simulink model "hexa_tilted_PID"  (R2023a)
settings: Solver=ode4  StartTime=0.0  StopTime=10  FixedStep=0.01  RelTol=1e-3
model workspace (MAT data in the model file):
  tf = Simulink.Parameter
  tf.Value = 60
  tf.DataType = 'auto'
  tf.Complexity = 'real'
  tf.Dimensions = [1 1]
  tray1 = [0  0  0  0  0  0; 0  0  0  0  0  0; 0  2  2  2  2  0; 0  0  0  0  0  0; 0  0  0  0  0  0; 0  0  0  0  0  0]
  tray2 = [0  2  2  -2  0  0; 0  -2  -2  2  0  0; 0  2  2  2  2  0; 0  0  0  0  0  0; 0  0  0  0  0  0; 0  0  0  0  0  0]
libraries: dspsrcs4 x6, simulink x3, robotcorelib x1
settings Model: Creator=adan  LastModifiedBy=adan
settings OptimizationCC: ReuseModelBlockBuffer=off

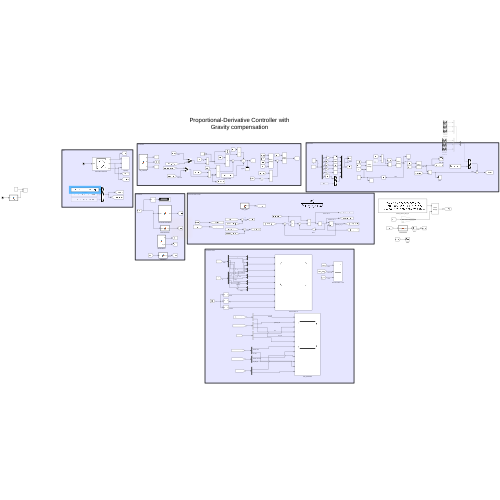
[thumbnail: Simulink's stored preview of the top-level diagram]
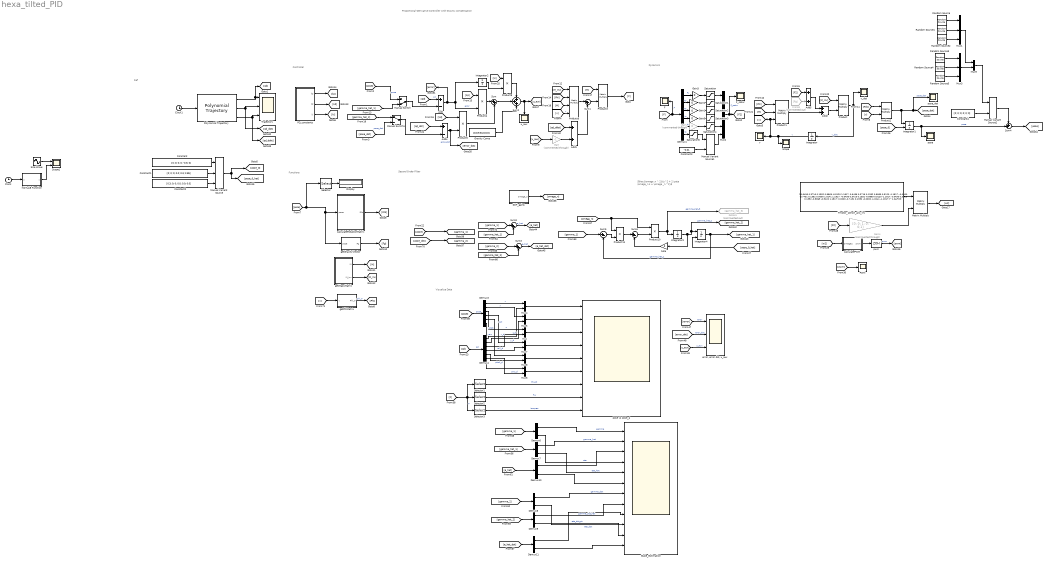
== system hexa_tilted_PID ==
  note: Ref
  note: Functions
  note: Second Order Filter
  note: Controller
  note: Visualize Data
  note: Dynamics
  note: Proportional-Derivative Controller with Gravity compensation
  note: $\frac{\omega_n ^ 2}{s^2 + 2 \zeta \omega_n s + \omega _n ^2}$
  Add : Sum  Inputs=+-
  Add1 : Sum
  Add2 : Sum
  Add4 : Sum  Inputs=+-
  Add5 : Sum
  Clock : Clock
  Clock1 : Clock
  Constant : Constant  Value=[0; 0; 0; 0; -0.3; 0]
  Constant1 : Constant  Value=[0; 0; 0; 0.0; 0.3; 2.85]
  Constant2 : Constant  Value=[0.3; 0; 0; 0.0; 0.0; 0.0]
  Constant3 : Constant  Value=-0.01
  Constant4 : Constant  Value=[0; 0; 0; 0; 0; 0]
  Demux1 : Demux  Outputs=6
  Demux{6..11} (6 alike) : Demux  Outputs=2
  Demux3 : Demux  Outputs=6
  Demux4 : Demux  Outputs=6
  Display : Display
  F : Scope
  F_satur : Scope
  From8 : From  Commented=on  GotoTag=Fg
  Gain : Gain  Commented=through  Gain=-1
  Gain{1..3,5} (4 alike) : Gain  Gain=0
  Gain4 : Gain  Commented=through  Gain=[0; 0; 1; 0; 0;1]
  Gain6 : Gain  Commented=through  Gain=0
  Goto41 : Goto  Commented=on  GotoTag=gamma_hat_3
  Gravity Comp : Constant  Value=[0;0;9.81;0;0;0]
  Integrator : Integrator  InitialCondition=[0; 0; 0; 0; 0; 0]
  Integrator1 : Integrator  InitialConditionSource=external  InitialCondition=[0; 0; 0; 0; 0; 0]
  Integrator2 : Integrator
  Integrator3 : Integrator
  Integrator4 : Integrator  InitialConditionSource=external
  MATLAB Function : MATLAB Function  TreatAsAtomicUnit=on
  Manual Variant Source : simulink/Signal Routing/Manual Variant Source  NumChoices=3  LabelModeActiveChoice=V_1
  Manual Variant Source1 : simulink/Signal Routing/Manual Variant Source  NumChoices=2  LabelModeActiveChoice=V_1
  Manual Variant Source2 : simulink/Signal Routing/Manual Variant Source  NumChoices=2  LabelModeActiveChoice=V_2
  Manual Switch : ManualSwitch  CurrentSetting=0
  Manual Switch1 : ManualSwitch
  Matrix Multiply : Product  Multiplication=Matrix(*)
  Mux{,4..9} (7 alike) : Mux  Inputs=2
  Mux1 : Mux  Inputs=3
  Mux2 : Mux  Inputs=6
  Mux3 : Mux  Inputs=3
  PD_constants : MATLAB Function  TreatAsAtomicUnit=on
  PWM : Scope
  Polynomial Trajectory : robotcorelib/Polynomial Trajectory  WaypointSource=Internal  Waypoints=zeros(6, 6)  TimePoints=[ 0, 5, 20, 28, 54, tf ]  TimeInterval=[ 1, 4 ]  Method=Cubic Polynomial  ParameterSource=Internal  VelocityBoundaryCondition=zeros( 6, 6 )  AccelerationBoundaryCondition=zeros( 2, 5 )  SimulateUsing=Interpreted execution
  Product : Product  Multiplication=Matrix(*)
  Product1 : Product  Inputs=3  Multiplication=Matrix(*)
  Product{4..5,8,10..11} (5 alike) : Product
  Product2 : Product  Multiplication=Matrix(*)
  Product3 : Product  Multiplication=Matrix(*)
  Product6 : Product  Inputs=4  Multiplication=Matrix(*)
  Random Source : dspsrcs4/Random Source  SrcType=Gaussian  NormMethod=Ziggurat  CltLength=12  MinVal=0  MaxVal=1  MeanVal=0.005  VarVal=0.001*0.001  RepMode=Not repeatable  rawSeed=1  IsInherit=off  SampMode=Discrete  SampTime=0.01  SampFrame=1  DataType=Double  OutComplex=Real  OutputFrames=off
  Random Source1 : dspsrcs4/Random Source  SrcType=Gaussian  NormMethod=Ziggurat  CltLength=12  MinVal=0  MaxVal=1  MeanVal=0.005  VarVal=0.001*0.001  RepMode=Not repeatable  rawSeed=1  IsInherit=off  SampMode=Discrete  SampTime=0.01  SampFrame=1  DataType=Double  OutComplex=Real  OutputFrames=off
  Random Source2 : dspsrcs4/Random Source  SrcType=Gaussian  NormMethod=Ziggurat  CltLength=12  MinVal=0  MaxVal=1  MeanVal=0.005  VarVal=0.001*0.001  RepMode=Not repeatable  rawSeed=1  IsInherit=off  SampMode=Discrete  SampTime=0.01  SampFrame=1  DataType=Double  OutComplex=Real  OutputFrames=off
  Random Source3 : dspsrcs4/Random Source  SrcType=Gaussian  NormMethod=Ziggurat  CltLength=12  MinVal=0  MaxVal=1  MeanVal=0.001  VarVal=0.001*0.001  RepMode=Not repeatable  rawSeed=1  IsInherit=off  SampMode=Discrete  SampTime=0.01  SampFrame=1  DataType=Double  OutComplex=Real  OutputFrames=off
  Random Source4 : dspsrcs4/Random Source  SrcType=Gaussian  NormMethod=Ziggurat  CltLength=12  MinVal=0  MaxVal=1  MeanVal=0.001  VarVal=0.001*0.001  RepMode=Not repeatable  rawSeed=1  IsInherit=off  SampMode=Discrete  SampTime=0.01  SampFrame=1  DataType=Double  OutComplex=Real  OutputFrames=off
  Random Source5 : dspsrcs4/Random Source  SrcType=Gaussian  NormMethod=Ziggurat  CltLength=12  MinVal=0  MaxVal=1  MeanVal=0.001  VarVal=0.001*0.001  RepMode=Not repeatable  rawSeed=1  IsInherit=off  SampMode=Discrete  SampTime=0.01  SampFrame=1  DataType=Double  OutComplex=Real  OutputFrames=off
  SOF_gains : MATLAB Function  TreatAsAtomicUnit=on
  Saturation : Saturate  UpperLimit=6  LowerLimit=-6
  Saturation1 : Saturate  UpperLimit=6  LowerLimit=-6
  Saturation2 : Saturate  UpperLimit=35  LowerLimit=0
  Saturation3 : Saturate
  Saturation4 : Saturate
  Saturation5 : Saturate
  Scope : Scope
  Scope1 : Scope  NumInputPorts=2
  Selector : Selector  InputPortWidth=6  IndexOptions=Index vector (dialog)  Indices=[4]  OutputSizes=1
  Selector1 : Selector  InputPortWidth=6  IndexOptions=Index vector (dialog)  Indices=[3]  OutputSizes=1
  Selector2 : Selector  InputPortWidth=6  IndexOptions=Index vector (dialog)  Indices=[1:2]  OutputSizes=1
  Selector3 : Selector  InputPortWidth=6  IndexOptions=Index vector (dialog)  Indices=[4:6]  OutputSizes=1
  Sine Wave : Sin  Amplitude=0.25  Frequency=0.5  SampleTime=0
  State_Estimation : Scope  NumInputPorts=12
  Sum : Sum  Inputs=|++
  Sum1 : Sum  Inputs=|-+
  Sum2 : Sum  Inputs=+++
  Sum{3,5..6,8} (4 alike) : Sum  Inputs=|+-
  Sum4 : Sum  Inputs=++|
  Tmotor_10inch_allo_inv : Constant  Value=|
      | [-0.6436    0.3716    0.1352    0.8869   -0.5120    1.1817;
      |             0.6436    0.3716    0.1352    0.8869    0.5120   -1.1817;
      |             -0.0000   -0.7431    0.1352    0.0000    1.0241    1.1817;
      |             -0.6436    0.3716    0.1352   -0.8869    0.5120   -1.1817;
      |             0.6436    0.3716    0.1352   -0.8869   -0.5120    1.1817;
      |             0.0000   -0.7431    0.1352   -0.0000   -1.0241   -1.1817;] * 1.0e+05;
  Trajectory : Scope  NumInputPorts=3
  calculatePWM : MATLAB Function  TreatAsAtomicUnit=on
  calculateRotationMatrix : MATLAB Function  TreatAsAtomicUnit=on
  "error, error dot, u_aux" : Scope  NumInputPorts=3
  getGravityVector : MATLAB Function  TreatAsAtomicUnit=on
  getMassMatrix : MATLAB Function  TreatAsAtomicUnit=on
  getPhiMatrix : MATLAB Function  TreatAsAtomicUnit=on
  pose : Scope
  pose vs pose_q : Scope  NumInputPorts=9
  pose_dot : Scope
  pwm : ZeroOrderHold  SampleTime=-1
  u_aux : Scope
  v : Scope
  v_dot : Scope
  zeta : Gain  Gain=2
  wires:
  Saturation/1 -> Mux2/1
  Saturation1/1 -> Mux2/2
  Saturation4/1 -> Mux2/5
  Saturation3/1 -> Mux2/4
  Demux1/6 -> Saturation5/1  "tz"
  Demux1/3 -> Gain1/1  "Fz"
  [F] -> F/1, Demux1/1  "F"
  Saturation5/1 -> Manual Variant Source1/1
  Demux1/2 -> Gain2/1  "Fy"
  Demux1/1 -> Gain3/1  "Fx"
  Demux1/5 -> Gain6/1  "ty"
  Demux1/4 -> Gain5/1  "tx"
  Saturation2/1 -> Mux2/3
  Mux2/1 -> F_satur/1, [F2]  "F_satur"
  [M] -> Product1/2
  [v] -> Product2/2
  [M_inv] -> Product/1
  Add2/1 -> Product/2
  Product/1 -> v_dot/1, Integrator/1  "v_dot"
  [Rib] -> Product2/1
  Product2/1 -> pose_dot/1, [pose_dot], Integrator1/1  "pose_dot"
  [Phi] -> Product1/1
  Product1/1 -> Add2/2
  Integrator1/1 -> pose/1, Sum4/2  "pose"
  Integrator/1 -> Scope/1, v/1, [v], Product1/3  "v"
  From8/1 -> Add5/2
  Add5/1 -> Add2/1
  [pose_dot] -> Manual Switch1/2  "pose_dot"
  [qd_dot] -> Add4/1
  [Phi] -> Product6/2
  Add4/1 -> [error_dot], Product5/2  "error_dot"
  [qd_ddot] -> Add1/1
  [qd] -> Add/1  "xd"
  [kp] -> Product4/1
  [v] -> Product6/4  "v"
  [kd] -> Product5/1
  Product4/1 -> Sum/1
  [M_inv] -> Product6/1
  [M] -> Product6/3
  Add/1 -> [error], Product4/2, Integrator2/1  "error"
  Product5/1 -> Sum/2
  [u_aux] -> Gain/1
  Sum2/1 -> [u_aux], u_aux/1
  [F2] -> Add5/1
  [ki] -> Product8/1
  Integrator2/1 -> Product8/2
  Gravity Comp/1 -> Sum2/3
  Sum/1 -> Sum2/2
  Product8/1 -> Sum2/1
  Add1/1 -> Sum1/2
  calculateRotationMatrix/1(Rib) -> [Rib]
  [pose] -> Selector/1, getGravityVector/1(pose), calculateRotationMatrix/1(pose)
  getGravityVector/1(Fg) -> [Fg]
  getPhiMatrix/1(Phi_T) -> [Phi]  "phi_T"
  Clock1/1 -> Polynomial Trajectory/1
  Polynomial Trajectory/2 -> Trajectory/2, [qd_dot]
  Polynomial Trajectory/3 -> Trajectory/3, [qd_ddot]
  Polynomial Trajectory/1 -> [qd], Trajectory/1
  Product6/1 -> Sum1/1
  Sum1/1 -> Product3/2
  [M] -> Product3/1
  Product3/1 -> [F]
  Demux3/5 -> Mux8/1  "pitch"
  Demux4/4 -> Mux7/2  "roll_d"
  Demux3/2 -> Mux5/1  "y"
  Mux5/1 -> pose vs pose_q/2
  Demux3/3 -> Mux/1  "z"
  [qd] -> Demux4/1  "qd"
  Mux8/1 -> pose vs pose_q/5
  Mux7/1 -> pose vs pose_q/4
  Mux4/1 -> pose vs pose_q/1
  Demux4/6 -> Mux6/2  "yaw_d"
  Demux4/1 -> Mux4/2  "x_d"
  Demux3/1 -> Mux4/1  "x"
  Demux3/4 -> Mux7/1  "roll"
  Mux6/1 -> pose vs pose_q/6
  [pose] -> Demux3/1  "pose"
  Mux/1 -> pose vs pose_q/3
  Demux4/5 -> Mux8/2  "pitch_d"
  Demux4/3 -> Mux/2  "z_d"
  Demux3/6 -> Mux6/1  "yaw"
  Demux4/2 -> Mux5/2  "y_d"
  [error_dot] -> "error, error dot, u_aux"/2  "error_dot"
  [error] -> "error, error dot, u_aux"/1  "error"
  [u_aux] -> "error, error dot, u_aux"/3  "u_aux"
  [gamma_hat_2] -> Demux9/1
  [gamma_hat_1] -> Demux7/1
  Demux6/2 -> State_Estimation/4  "eta"
  Demux7/2 -> State_Estimation/5  "eta_hat"
  Demux8/2 -> State_Estimation/10  "eta_dot"
  [gamma_2] -> Sum3/1
  [gamma_2] -> Demux8/1
  [omega_n] -> Product11/1, Product10/1
  [gamma_1] -> Demux6/1
  [e_hat_dot] -> Demux11/1
  Demux8/1 -> State_Estimation/7  "gamma_dot"
  SOF_gains/1(omega_n) -> [omega_n]
  [gamma_hat_2] -> Sum3/2
  [gamma_1] -> Sum8/1
  Demux11/1 -> State_Estimation/9
  Integrator3/1 -> zeta/1, [gamma_hat_2], Integrator4/1  "gamma_hat_2"
  Demux6/1 -> State_Estimation/1  "gamma"
  [gamma_1] -> Sum5/1
  Demux9/2 -> State_Estimation/11  "eta_dot_at"
  zeta/1 -> Sum6/2
  Demux11/2 -> State_Estimation/12
  Demux10/2 -> State_Estimation/6
  [e_hat] -> Demux10/1
  Demux7/1 -> State_Estimation/2  "gamma_hat"
  Demux10/1 -> State_Estimation/3
  Sum6/1 -> Product10/2
  Sum3/1 -> [e_hat_dot]  "e_hat"
  Integrator4/1 -> Sum5/2, [gamma_hat_1]  "gamma_hat_1"
  Sum5/1 -> Product11/2
  [gamma_hat_1] -> Sum8/2
  Sum8/1 -> [e_hat]  "e_hat"
  Product10/1 -> Integrator3/1, Goto41/1  "gamma_hat_3"
  Product11/1 -> Sum6/1
  Demux9/1 -> State_Estimation/8  "gamma_dot_hat"
  [pose] -> [gamma_1]
  [pose_dot] -> [gamma_2]
  PD_constants/3(ki) -> [ki]
  [v] -> getPhiMatrix/1(v)
  getMassMatrix/2(M_inv) -> [M_inv]
  getMassMatrix/1(M) -> [M]
  Gain/1 -> Add1/2
  [pose] -> Manual Switch/1  "pose"
  [gamma_hat_1] -> Manual Switch/2
  Manual Switch/1 -> Add/2
  [gamma_hat_2] -> Manual Switch1/1
  Manual Switch1/1 -> Add4/2
  Selector/1 -> Display/1
  Constant/1 -> Manual Variant Source/1
  Constant1/1 -> Manual Variant Source/2
  Manual Variant Source/1 -> [pose_0], [pose_0_hat]
  [pose_0] -> Integrator1/2
  [pose_0_hat] -> Integrator4/2
  [F] -> Selector1/1, Selector3/1, Selector2/1  "F"
  Selector1/1 -> pose vs pose_q/7  "thrust"
  Selector2/1 -> pose vs pose_q/8  "fxy"
  Selector3/1 -> pose vs pose_q/9  "torques"
  PD_constants/1(kp) -> [kp]
  PD_constants/2(kd) -> [kd]
  Constant2/1 -> Manual Variant Source/3
  Gain1/1 -> Saturation2/1
  Gain2/1 -> Saturation1/1
  Gain3/1 -> Saturation/1
  Tmotor_10inch_allo_inv/1 -> Matrix Multiply/1
  [F2] -> Gain4/1
  calculatePWM/1(pwm) -> pwm/1
  [w2] -> calculatePWM/1(omega2)
  [pwm] -> PWM/1
  pwm/1 -> [pwm]  "pwm"
  Matrix Multiply/1 -> [w2]
  Gain4/1 -> Matrix Multiply/2
  Gain5/1 -> Saturation3/1
  Gain6/1 -> Saturation4/1
  Manual Variant Source1/1 -> Mux2/6
  Constant3/1 -> Manual Variant Source1/2
  Sine Wave/1 -> Scope1/1
  Clock/1 -> MATLAB Function/1(u)
  MATLAB Function/1(y) -> Scope1/2
  Sum4/1 -> [pose]
  Manual Variant Source2/1 -> Sum4/1
  Constant4/1 -> Manual Variant Source2/2
  Random Source/1 -> Mux1/1
  Random Source2/1 -> Mux1/3
  Random Source1/1 -> Mux1/2
  Random Source4/1 -> Mux3/2
  Random Source5/1 -> Mux3/3
  Random Source3/1 -> Mux3/1
  Mux3/1 -> Mux9/2
  Mux1/1 -> Mux9/1
  Mux9/1 -> Manual Variant Source2/1

== matlab function hexa_tilted_PID/getPhiMatrix ==
  data: v input; Phi_T output
function Phi_T = fcn(v)

%% Phi matrix calculation
uu = v(1);
vv = v(2);
ww = v(3);
pp = v(4);
qq = v(5);
rr = v(6);


Phi = [0, -rr, qq, 0, -ww, vv;
        rr, 0, -pp , ww, 0, -uu;
        -qq, pp, 0,  -vv, uu, 0;
        0, 0, 0, 0, -rr, qq; 
        0, 0, 0, rr, 0, -pp;
        0, 0, 0, -qq, pp, 0];

Phi_T = Phi;

== matlab function hexa_tilted_PID/PD_constants ==
  data: kp output; kd output; ki output
function [kp, kd, ki] = fcn

%% Buenas ganancias
% kp = [3.5; 3.5; 3; 1.1; 1.1; 0.85];
% kd = [3.25; 3.25; 3; 1.75; 1.75; 1.5];

%% Ganancias lentas
kp = [0.1; 0.1; 0.01; 0.05; 2; 2];
kd = [0.5; 0.5; 0.2; 0.5; 2; 2];
ki = [0; 0; 0; 0; 0; 0];

== matlab function hexa_tilted_PID/calculateRotationMatrix ==
  data: Rib output; pose input
function Rib  = fcn(pose)

roll = pose(4);
pitch = pose(5);
yaw = pose(6);

R1 = [cos(yaw)*cos(pitch), -cos(roll)*sin(yaw) + cos(yaw)*sin(roll)*sin(pitch), sin(roll)*sin(yaw) + cos(roll)*cos(yaw)*sin(pitch);
       cos(pitch)*sin(yaw), cos(roll)*cos(yaw) + sin(yaw)*sin(pitch)*sin(roll), -cos(yaw)*sin(roll) + sin(yaw)*sin(pitch)*cos(roll);
       -sin(pitch), cos(pitch)*sin(roll), cos(pitch)*cos(roll)];

R2 = [1, sin(roll)*tan(pitch), cos(roll)*tan(pitch);
      0, cos(roll), -sin(roll);
      0, sin(roll)/cos(pitch), cos(roll)/cos(pitch)];

Rzeros = zeros(3);

Rib = [R1, Rzeros;
       Rzeros, R2];

== matlab function hexa_tilted_PID/getMassMatrix ==
  data: M output; M_inv output
function [M, M_inv] = fcn

m = 1.8;
Jxx = 0.0374;
Jyy = 0.0385;
Jzz = 0.0593;

M = [m, 0, 0, 0, 0, 0;
    0, m, 0, 0, 0, 0;
    0, 0, m, 0, 0, 0;
    0, 0, 0, Jxx, 0, 0;
    0, 0, 0, 0, Jyy, 0;
    0, 0, 0, 0, 0, Jzz];

M_inv = inv(M);

== matlab function hexa_tilted_PID/getGravityVector ==
  data: Fg output; pose input
function Fg = fcn(pose)

roll = pose(4);
pitch = pose(5);

%% Fg matrix calculation

m = 1.8;
g = 9.81;

Fg = [m*g*sin(pitch);
      -m*g*cos(pitch)*sin(roll);
      -m*g*cos(pitch)*cos(roll);
      0;
      0;
      0];

== matlab function hexa_tilted_PID/calculatePWM ==
  data: omega2 input; pwm output
function pwm = fcn(omega2)

pwm = -1.3121e-09 .* omega2 .* omega2 + 0.00208 .* omega2 + 1107.922;

== matlab function hexa_tilted_PID/MATLAB Function ==
  data: u input; y output
function y = fcn(u)

y = 0.25 * sin(0.5 * u);

== matlab function hexa_tilted_PID/SOF_gains ==
  data: omega_n output
function omega_n = fcn

omega_n = [30; 30; 50; 20; 20; 20];
